simulink model "BiCopter_Control_V3"  (R2022a)
settings: Solver=VariableStepAuto  StartTime=0.0  StopTime=10  RelTol=1e-3
values from neighbouring files (symbols this model uses):
  At = [0 1; 0 0]    [BiCopter_V0.m]    (also in BiCopter_runner.m)
  Bt = [0;1/J]    [BiCopter_V0.m]    (also in BiCopter_runner.m)
  C = [eye(2) zeros(2)]    [BiCopter_V0.m]    (also in BiCopter_runner.m)
  C12_IL = I12([8 11],:)    [BiCopter_V0.m]    (also in BiCopter_runner.m = I12(5:6,:))
  C12_OL = I12([1 3 4 6],:)    [BiCopter_V0.m]    (also in BiCopter_runner.m = I12(1:4,:))
  Ct = [1 0]    [BiCopter_V0.m]    (also in BiCopter_runner.m)
  J = 3    [BiCopter_V0.m]    (also in BiCopter_runner.m)
  Kq = Ka(:,5:6)    [BiCopter_V0.m]    (also in BiCopter_runner.m)
  Ktq = Kta(:,3)    [BiCopter_V0.m]    (also in BiCopter_runner.m)
  Ktx = Kta(:,1:2)    [BiCopter_V0.m]    (also in BiCopter_runner.m)
  Kx = Ka(:,1:4)    [BiCopter_V0.m]    (also in BiCopter_runner.m)
  m = 2    [BiCopter_V0.m]    (also in BiCopter_runner.m)
  theta_r = rand(1,1)    [BiCopter_V0.m]    (also in BiCopter_runner.m)
  x_r = rand(2,1)    [BiCopter_V0.m]    (also in BiCopter_runner.m = randn(2,1))
settings Model: Creator=Ankit  LastModifiedBy=Ankit

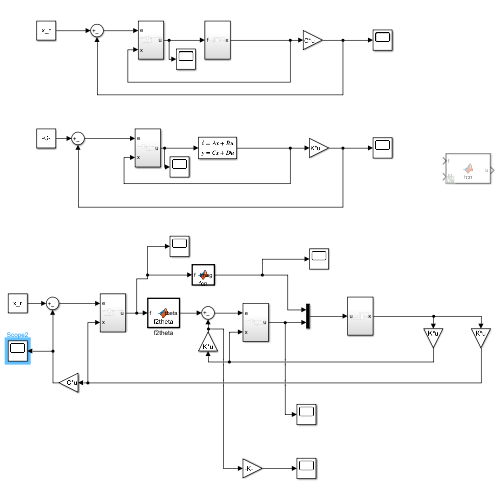
[thumbnail: Simulink's stored preview of the top-level diagram]
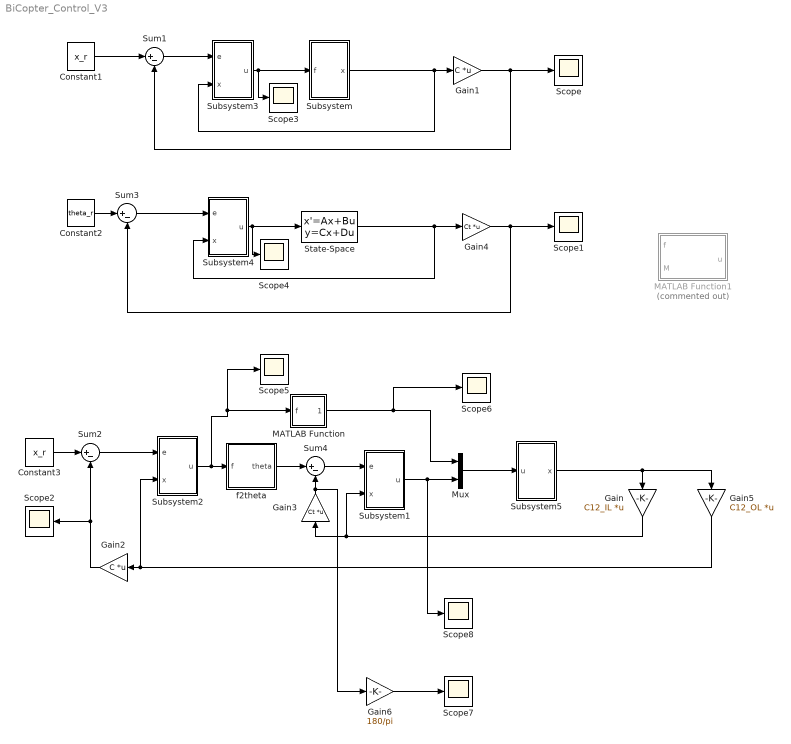
== system BiCopter_Control_V3 ==
  Constant1 : Constant  Value=x_r
  Constant2 : Constant  Value=theta_r
  Constant3 : Constant  Value=x_r
  Gain : Gain  Gain=C12_IL  Multiplication=Matrix(K*u)
  Gain1 : Gain  Gain=C  Multiplication=Matrix(K*u)
  Gain2 : Gain  Gain=C  Multiplication=Matrix(K*u)
  Gain3 : Gain  Gain=Ct  Multiplication=Matrix(K*u)
  Gain4 : Gain  Gain=Ct  Multiplication=Matrix(K*u)
  Gain5 : Gain  Gain=C12_OL  Multiplication=Matrix(K*u)
  Gain6 : Gain  Gain=180/pi
  MATLAB Function : MATLAB Function  TreatAsAtomicUnit=on
  MATLAB Function1 : MATLAB Function  Commented=on  TreatAsAtomicUnit=on
  Mux : Mux  Inputs=2
  Scope{,1..8} (9 alike) : Scope
  State-Space : StateSpace  A=At  B=Bt  C=eye(2)  D=zeros(2,1)  InitialCondition=0
  Subsystem : Subsystem
  Subsystem1 : Subsystem
  Subsystem2 : Subsystem
  Subsystem3 : Subsystem
  Subsystem4 : Subsystem
  Subsystem5 : Subsystem
  Sum{1..4} (4 alike) : Sum  Inputs=|+-
  f2theta : MATLAB Function  TreatAsAtomicUnit=on
  wires:
  Gain1/1 -> Scope/1, Sum1/2
  Constant1/1 -> Sum1/1
  Subsystem/1(x) -> Gain1/1, Subsystem3/2(x)
  Gain4/1 -> Scope1/1, Sum3/2
  State-Space/1 -> Gain4/1, Subsystem4/2(x)
  Constant2/1 -> Sum3/1
  Sum1/1 -> Subsystem3/1(e)
  Subsystem3/1(u) -> Scope3/1, Subsystem/1(f)
  Sum3/1 -> Subsystem4/1(e)
  Subsystem4/1(u) -> Scope4/1, State-Space/1
  Sum2/1 -> Subsystem2/1(e)
  Gain2/1 -> Scope2/1, Sum2/2
  Constant3/1 -> Sum2/1
  Sum4/1 -> Subsystem1/1(e)
  Gain3/1 -> Gain6/1, Sum4/2
  Gain/1 -> Subsystem1/2(x), Gain3/1
  Gain5/1 -> Subsystem2/2(x), Gain2/1
  Subsystem2/1(u) -> MATLAB Function/1(f), Scope5/1, f2theta/1(f)
  Subsystem1/1(u) -> Scope8/1, Mux/2
  Subsystem5/1(x) -> Gain5/1, Gain/1
  MATLAB Function/1(fmag) -> Mux/1, Scope6/1
  Mux/1 -> Subsystem5/1(u)
  f2theta/1(theta) -> Sum4/1
  Gain6/1 -> Scope7/1

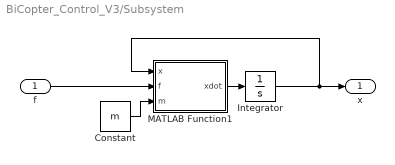
== system BiCopter_Control_V3/Subsystem ==
  f : Inport
  Constant : Constant  Value=m
  Integrator : Integrator
  MATLAB Function1 : MATLAB Function  TreatAsAtomicUnit=on
  x : Outport
  wires:
  Constant/1 -> MATLAB Function1/3(m)
  MATLAB Function1/1(xdot) -> Integrator/1
  f/1 -> MATLAB Function1/2(f)
  Integrator/1 -> MATLAB Function1/1(x), x/1

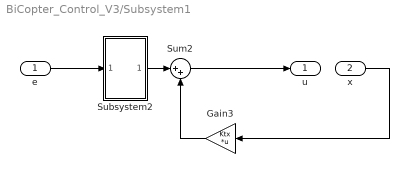
== system BiCopter_Control_V3/Subsystem1 ==
  e : Inport
  x : Inport  Port=2
  Gain3 : Gain  Gain=Ktx  Multiplication=Matrix(K*u)
  Subsystem2 : Subsystem
  Sum2 : Sum  Inputs=|++
  u : Outport
  wires:
  Subsystem2/1(Out1) -> Sum2/1
  Gain3/1 -> Sum2/2
  Sum2/1 -> u/1
  e/1 -> Subsystem2/1(In1)
  x/1 -> Gain3/1

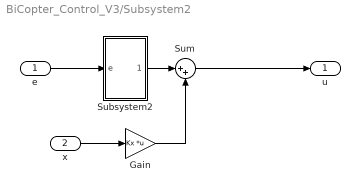
== system BiCopter_Control_V3/Subsystem2 ==
  e : Inport
  x : Inport  Port=2
  Gain : Gain  Gain=Kx  Multiplication=Matrix(K*u)
  Subsystem2 : Subsystem
  Sum : Sum  Inputs=|++
  u : Outport
  wires:
  e/1 -> Subsystem2/1(e)
  Gain/1 -> Sum/2
  Subsystem2/1(u_int) -> Sum/1
  x/1 -> Gain/1
  Sum/1 -> u/1

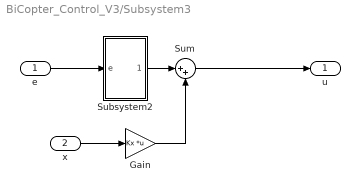
== system BiCopter_Control_V3/Subsystem3 ==
  e : Inport
  x : Inport  Port=2
  Gain : Gain  Gain=Kx  Multiplication=Matrix(K*u)
  Subsystem2 : Subsystem
  Sum : Sum  Inputs=|++
  u : Outport
  wires:
  e/1 -> Subsystem2/1(e)
  Gain/1 -> Sum/2
  Subsystem2/1(u_int) -> Sum/1
  x/1 -> Gain/1
  Sum/1 -> u/1

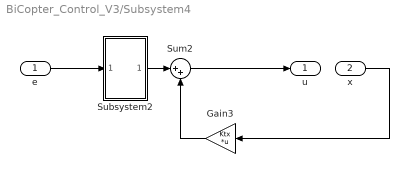
== system BiCopter_Control_V3/Subsystem4 ==
  e : Inport
  x : Inport  Port=2
  Gain3 : Gain  Gain=Ktx  Multiplication=Matrix(K*u)
  Subsystem2 : Subsystem
  Sum2 : Sum  Inputs=|++
  u : Outport
  wires:
  Subsystem2/1(Out1) -> Sum2/1
  Gain3/1 -> Sum2/2
  Sum2/1 -> u/1
  e/1 -> Subsystem2/1(In1)
  x/1 -> Gain3/1

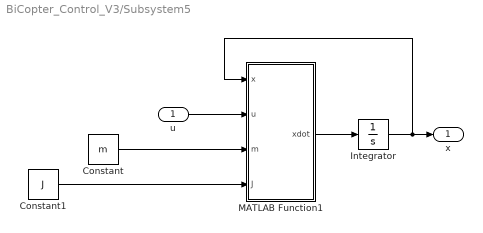
== system BiCopter_Control_V3/Subsystem5 ==
  u : Inport
  Constant : Constant  Value=m
  Constant1 : Constant  Value=J
  Integrator : Integrator
  MATLAB Function1 : MATLAB Function  TreatAsAtomicUnit=on
  x : Outport
  wires:
  Constant/1 -> MATLAB Function1/3(m)
  MATLAB Function1/1(xdot) -> Integrator/1
  u/1 -> MATLAB Function1/2(u)
  Integrator/1 -> MATLAB Function1/1(x), x/1
  Constant1/1 -> MATLAB Function1/4(J)

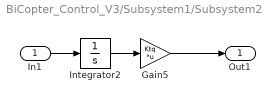
== system BiCopter_Control_V3/Subsystem1/Subsystem2 ==
  In1 : Inport
  Gain5 : Gain  Gain=Ktq  Multiplication=Matrix(K*u)
  Integrator2 : Integrator
  Out1 : Outport
  wires:
  Integrator2/1 -> Gain5/1
  Gain5/1 -> Out1/1
  In1/1 -> Integrator2/1

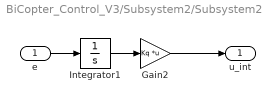
== system BiCopter_Control_V3/Subsystem2/Subsystem2 ==
  e : Inport
  Gain2 : Gain  Gain=Kq  Multiplication=Matrix(K*u)
  Integrator1 : Integrator
  u_int : Outport
  wires:
  Integrator1/1 -> Gain2/1
  Gain2/1 -> u_int/1
  e/1 -> Integrator1/1

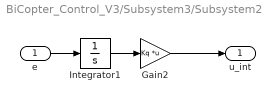
== system BiCopter_Control_V3/Subsystem3/Subsystem2 ==
  e : Inport
  Gain2 : Gain  Gain=Kq  Multiplication=Matrix(K*u)
  Integrator1 : Integrator
  u_int : Outport
  wires:
  Integrator1/1 -> Gain2/1
  Gain2/1 -> u_int/1
  e/1 -> Integrator1/1

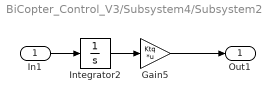
== system BiCopter_Control_V3/Subsystem4/Subsystem2 ==
  In1 : Inport
  Gain5 : Gain  Gain=Ktq  Multiplication=Matrix(K*u)
  Integrator2 : Integrator
  Out1 : Outport
  wires:
  Integrator2/1 -> Gain5/1
  Gain5/1 -> Out1/1
  In1/1 -> Integrator2/1

== matlab function BiCopter_Control_V3/Subsystem/MATLAB Function1 ==
  data: x input; xdot output; f input; m input
function xdot = fcn(x,f,m)

xdot = zeros(4,1);

xdot(1:2,1) = x(3:4,1);

xdot(3:4,1) = f/m+[0;10];

end

== matlab function BiCopter_Control_V3/MATLAB Function ==
  data: f input; fmag output
function fmag = fcn(f)

fmag = sqrt(f(1)^2+f(2)^2); % sqrt(f'*f);

== matlab function BiCopter_Control_V3/f2theta ==
  data: f input; theta output
function theta = f2theta(f)

theta = 0;

theta = atan2(-f(1),-f(2));

== matlab function BiCopter_Control_V3/MATLAB Function1 ==
  data: f input; u output; M input
function u = fcn(f, M)

u = zeros(4,1);
u(1) = norm(f);

u(2) = M;

== matlab function BiCopter_Control_V3/Subsystem5/MATLAB Function1 ==
  data: x input; xdot output; u input; m input; J input
function xdot = fcn(x,u,m,J)

xdot = zeros(6,1);

xdot(1:2,1) = x(3:4,1);
xdot(5,1)   = x(6,1);


theta = x(5);

xdot(3:4,1) = -u(1)/m*[sin(theta); cos(theta)]+[0;10];



xdot(6,1)   = u(2)/J;






end
